simulink model "compact_anf"  (R2017b)
settings: Solver=VariableStepAuto  StartTime=0.0  StopTime=0.2  MaxStep=1e-4  RelTol=1e-3
libraries: powerlib x5, peSinusoidalMeasurement x1
settings Model: Creator=Kalpit  LastModifiedBy=Kalpit

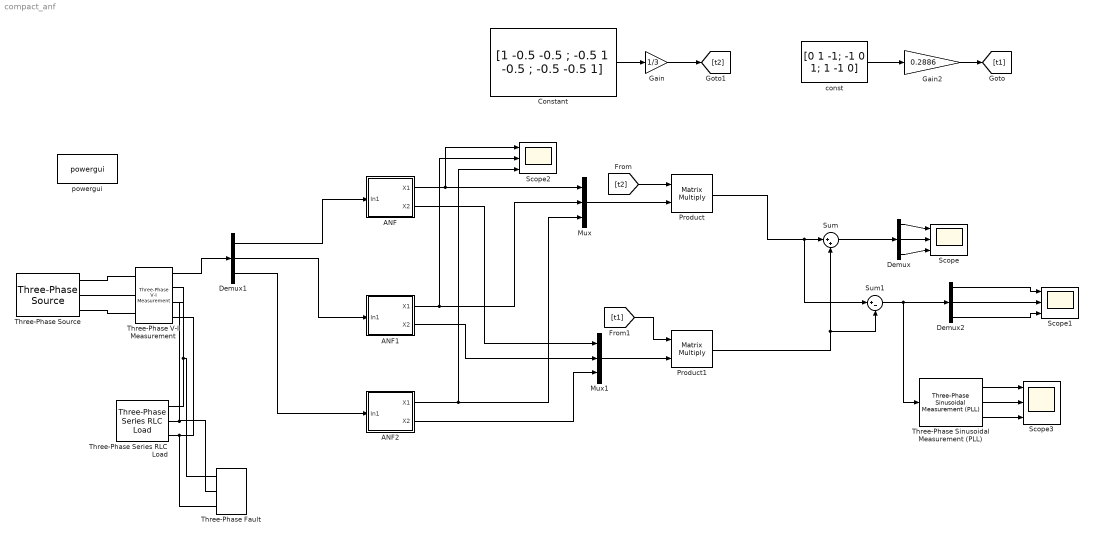
== system compact_anf ==
  ANF : Subsystem
  ANF1 : Subsystem
  ANF2 : Subsystem
  Constant : Constant  Value=[1 -0.5 -0.5 ; -0.5 1 -0.5 ; -0.5 -0.5 1]
  Demux : Demux  Outputs=3
  Demux1 : Demux  Outputs=3
  Demux2 : Demux  Outputs=3
  Gain : Gain  Gain=1/3
  Gain2 : Gain  Gain=0.2886
  Mux : Mux  Inputs=3
  Mux1 : Mux  Inputs=3
  Product : Product  Multiplication=Matrix(*)
  Product1 : Product  Multiplication=Matrix(*)
  Scope{,1..3} (4 alike) : Scope  NumInputPorts=3
  Sum : Sum  Inputs=|++
  Sum1 : Sum  Inputs=|+-
  Three-Phase Series RLC Load : powerlib/Elements/Three-Phase Series RLC Load  LConnTagsString=A|B|C  Configuration=Y (grounded)  NominalVoltage=415  Vabc=[1e3 1e3 1e3]  Vabcp=[1e3 1e3 1e3]  NominalFrequency=50  UnbalancedPower=off  ActivePower=10e3  InductivePower=100  CapacitivePower=100  Pabc=[10e3 9e3 11e3]  QLabc=[100 90 110]  QCabc=[100 90 110]  Pabcp=[10e3 9e3 11e3]  QLabcp=[100 90 110]  QCabcp=[100 90 110]  Measurements=None  LoadType=constant Z
  Three-Phase V-I Measurement : powerlib/Measurements/Three-Phase V-I Measurement  VoltageMeasurement=phase-to-ground  SetLabelV=off  LabelV=Vabc  Vpu=off  VpuLL=off  CurrentMeasurement=no  SetLabelI=off  LabelI=Iabc  Ipu=off  Pbase=100e6  Vbase=1  OutputType=Complex  PhasorSimulation=off  PSBequivalent=0
  Three-Phase Fault : powerlib/Elements/Three-Phase Fault  InitialStates=0  FaultA=on  FaultB=off  FaultC=on  GroundFault=on  SwitchTimes=0.2  External=off  SwitchStatus=NaN  FaultResistance=0.001  GroundResistance=0.01  SnubberResistance=1e6  SnubberCapacitance=inf  Measurements=None
  Three-Phase Sinusoidal Measurement (PLL) : peSinusoidalMeasurement/Three-Phase Sinusoidal Measurement (PLL)  Kp_LF=200  Ki_LF=2000  F0=60  Theta0=0  Ts=-1
  Three-Phase Source : powerlib/Electrical Sources/Three-Phase Source  InternalConnection=Yg  VoltagePhases=off  Voltage=415  PhaseAngle=0  Voltage_phases=[25e3 25e3 25e3]/sqrt(3)  PhaseAngles_phases=[0 -120 +120]  Frequency=50  NonIdealSource=on  SpecifyImpedance=off  Resistance=0.8929  Inductance=16.58e-3  ShortCircuitLevel=100e6  BaseVoltage=25e3  XRratio=7  BusType=swing  Pref=10e3  Qref=0  Prefabc=[10e3, 10e3, 10e3]  Qrefabc=[0, 0, 0]  Qmin=-inf  Qmax=inf
  const : Constant  Value=[0 1 -1; -1 0 1; 1 -1 0]
  powergui : powerlib/powergui  Priority=1  SimulationMode=Continuous  SampleTime=50e-6  frequency=60  Iterations=50  frequencyindice=50  Pbase=100e6  ErrMax=1e-4  UnitsV=kV  UnitsW=MW  buscounter=0  FunctionMessages=off  echomessages=off  EnableUseOfTLC=off  CurrentSourceSwitches=off  DisableSnubberDevices=off  DisableRonSwitches=off  DisableVfSwitches=off  DisplayEquations=off  SolverType=Tustin/Backward Euler (TBE)  Interpol=off  ExternalGateDelay=off  methode=off  Ts=100  x0status=blocks  SPID=on  SwTol=0  HookPort=off  RestoreLinks=warning  ResistiveCurrentMeasurement=off  Frange=[0:2:500]  Ylog=off  Xlog=on  ShowGrid=off  save=off  variable=ZData  structure=0  ZoomFFT=off  StartTime=0.0  cycles=1  DisplayStyle=1  fundamental=60  FreqAxis=off  MaxFrequency=1000  frequencyindicesteady=1  RmsSteady=1  display=off
  wires:
  ANF/1(X1) -> Scope2/1, Mux/1
  ANF1/1(X1) -> Scope2/2, Mux/2
  ANF2/1(X1) -> Scope2/3, Mux/3
  ANF/2(X2) -> Mux1/1
  ANF1/2(X2) -> Mux1/2
  ANF2/2(X2) -> Mux1/3
  Gain2/1 -> [t1]
  const/1 -> Gain2/1
  Constant/1 -> Gain/1
  Gain/1 -> [t2]
  Mux/1 -> Product/2
  Mux1/1 -> Product1/2
  [t2] -> Product/1
  [t1] -> Product1/1
  Product/1 -> Sum1/1, Sum/1
  Product1/1 -> Sum1/2, Sum/2
  Sum/1 -> Demux/1
  Demux/3 -> Scope/3
  Demux/2 -> Scope/2
  Demux/1 -> Scope/1
  Three-Phase V-I Measurement/1 -> Demux1/1
  Demux1/1 -> ANF/1(In1)
  Demux1/2 -> ANF1/1(In1)
  Demux1/3 -> ANF2/1(In1)
  Demux2/1 -> Scope1/1
  Demux2/2 -> Scope1/2
  Sum1/1 -> Three-Phase Sinusoidal Measurement (PLL)/1, Demux2/1
  Demux2/3 -> Scope1/3
  Three-Phase Sinusoidal Measurement (PLL)/3 -> Scope3/3
  Three-Phase Sinusoidal Measurement (PLL)/2 -> Scope3/2
  Three-Phase Sinusoidal Measurement (PLL)/1 -> Scope3/1
  connections:
  Three-Phase V-I Measurement/RConn3 -- Three-Phase Fault/LConn3 -- Three-Phase Series RLC Load/LConn3
  Three-Phase Series RLC Load/LConn1 -- Three-Phase Fault/LConn1 -- Three-Phase V-I Measurement/RConn1
  Three-Phase Series RLC Load/LConn2 -- Three-Phase V-I Measurement/RConn2 -- Three-Phase Fault/LConn2
  Three-Phase Source/RConn1 -- Three-Phase V-I Measurement/LConn1
  Three-Phase Source/RConn3 -- Three-Phase V-I Measurement/LConn3
  Three-Phase V-I Measurement/LConn2 -- Three-Phase Source/RConn2

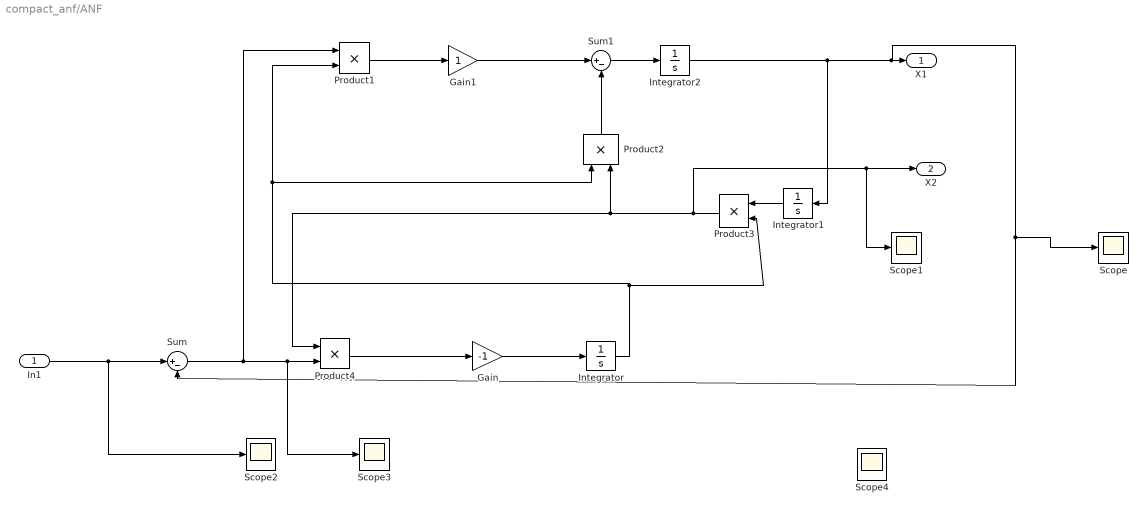
== system compact_anf/ANF ==
  In1 : Inport
  Gain : Gain  Gain=-1
  Gain1 : Gain
  Integrator : Integrator  InitialCondition=100*pi
  Integrator1 : Integrator
  Integrator2 : Integrator
  Product{1..4} (4 alike) : Product
  Scope{,1..4} (5 alike) : Scope
  Sum : Sum  Inputs=|+-
  Sum1 : Sum  Inputs=|+-
  X1 : Outport
  X2 : Outport  Port=2
  wires:
  Sum1/1 -> Integrator2/1
  Sum/1 -> Product1/1, Scope3/1, Product4/2
  Product4/1 -> Gain/1
  In1/1 -> Scope2/1, Sum/1
  Integrator1/1 -> Product3/1
  Integrator2/1 -> Scope/1, Sum/2, X1/1, Integrator1/1
  Integrator/1 -> Product3/2, Product2/1, Product1/2
  Product3/1 -> Scope1/1, X2/1, Product4/1, Product2/2
  Product1/1 -> Gain1/1
  Product2/1 -> Sum1/2
  Gain/1 -> Integrator/1
  Gain1/1 -> Sum1/1

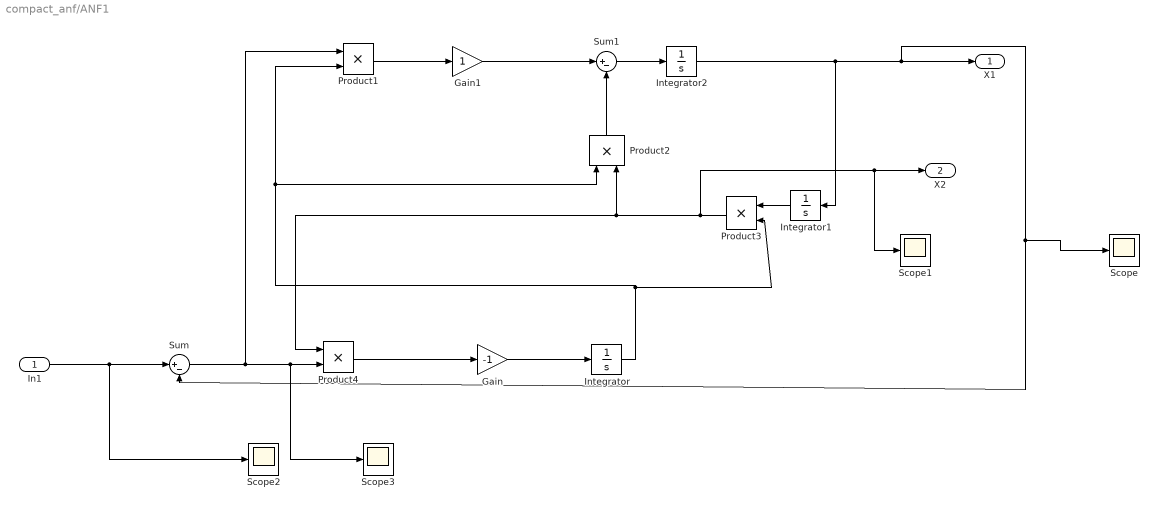
== system compact_anf/ANF1 ==
  In1 : Inport
  Gain : Gain  Gain=-1
  Gain1 : Gain
  Integrator : Integrator  InitialCondition=100*pi
  Integrator1 : Integrator
  Integrator2 : Integrator
  Product{1..4} (4 alike) : Product
  Scope{,1..3} (4 alike) : Scope
  Sum : Sum  Inputs=|+-
  Sum1 : Sum  Inputs=|+-
  X1 : Outport
  X2 : Outport  Port=2
  wires:
  Gain1/1 -> Sum1/1
  Gain/1 -> Integrator/1
  Product2/1 -> Sum1/2
  Product1/1 -> Gain1/1
  Product3/1 -> Product2/2, Product4/1, X2/1, Scope1/1
  Integrator/1 -> Product1/2, Product2/1, Product3/2
  Integrator2/1 -> Integrator1/1, X1/1, Sum/2, Scope/1
  Integrator1/1 -> Product3/1
  In1/1 -> Sum/1, Scope2/1
  Product4/1 -> Gain/1
  Sum/1 -> Product4/2, Scope3/1, Product1/1
  Sum1/1 -> Integrator2/1

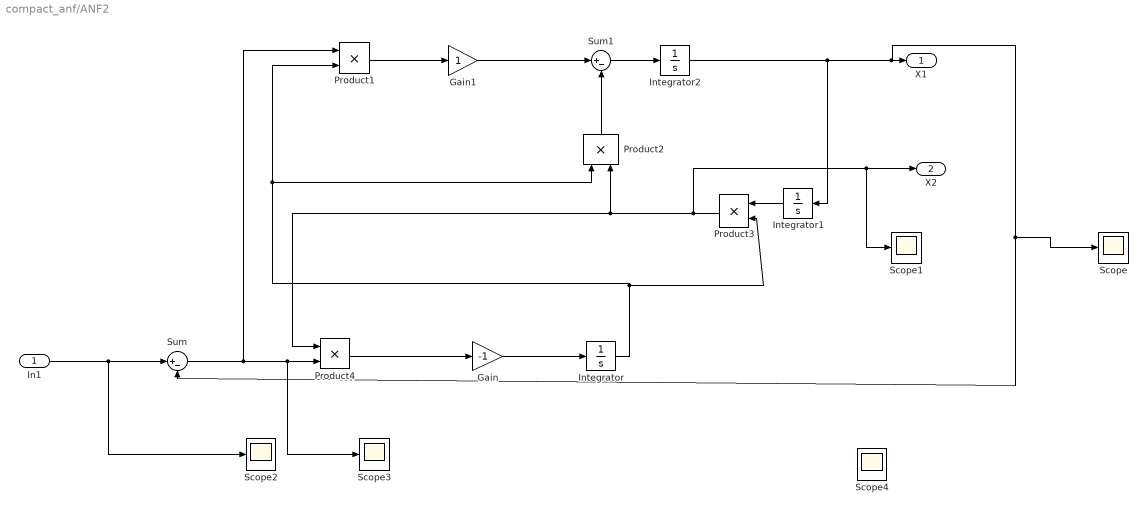
== system compact_anf/ANF2 ==
  In1 : Inport
  Gain : Gain  Gain=-1
  Gain1 : Gain
  Integrator : Integrator  InitialCondition=100*pi
  Integrator1 : Integrator
  Integrator2 : Integrator
  Product{1..4} (4 alike) : Product
  Scope{,1..4} (5 alike) : Scope
  Sum : Sum  Inputs=|+-
  Sum1 : Sum  Inputs=|+-
  X1 : Outport
  X2 : Outport  Port=2
  wires:
  Sum1/1 -> Integrator2/1
  Sum/1 -> Product1/1, Scope3/1, Product4/2
  Product4/1 -> Gain/1
  In1/1 -> Scope2/1, Sum/1
  Integrator1/1 -> Product3/1
  Integrator2/1 -> Scope/1, Sum/2, X1/1, Integrator1/1
  Integrator/1 -> Product3/2, Product2/1, Product1/2
  Product3/1 -> Scope1/1, X2/1, Product4/1, Product2/2
  Product1/1 -> Gain1/1
  Product2/1 -> Sum1/2
  Gain/1 -> Integrator/1
  Gain1/1 -> Sum1/1
